simulink model "ForwardKinematicsSim2"  (R2020a)
settings: Solver=VariableStepAuto  StartTime=0.0  StopTime=10.0  RelTol=1e-3
settings Model: Creator=Sheldon  LastModifiedBy=alan

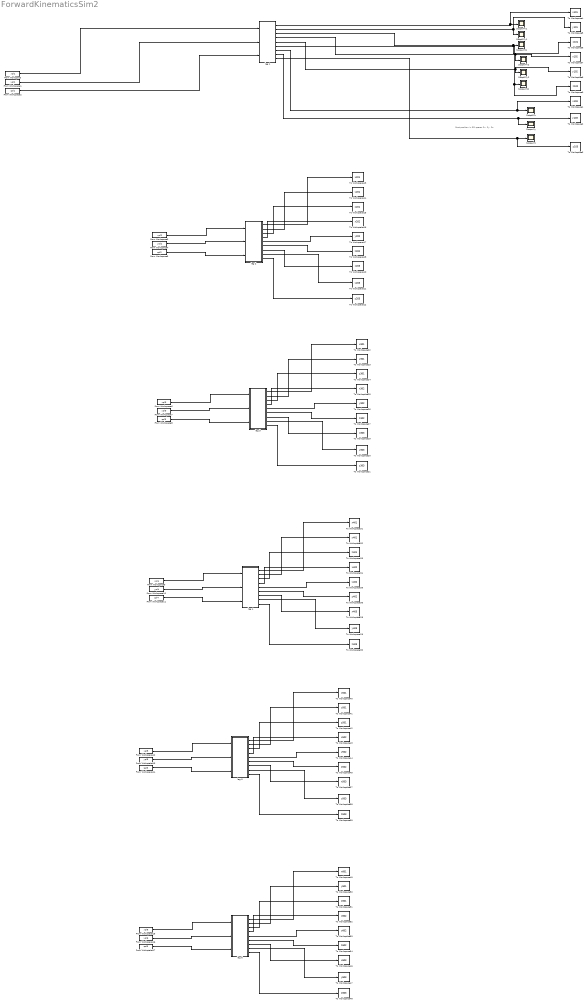
== system ForwardKinematicsSim2 ==
  note: Foot position in 3D space:
      | Px, Py, Pz
  From Workspace : FromWorkspace  VariableName=xpl1  SampleTime=1
  From Workspace1 : FromWorkspace  VariableName=ypl1  SampleTime=1
  From Workspace10 : FromWorkspace  VariableName=ypl4  SampleTime=1
  From Workspace11 : FromWorkspace  VariableName=zpl4  SampleTime=1
  From Workspace12 : FromWorkspace  VariableName=xpl5  SampleTime=1
  From Workspace13 : FromWorkspace  VariableName=ypl5  SampleTime=1
  From Workspace14 : FromWorkspace  VariableName=zpl5  SampleTime=1
  From Workspace15 : FromWorkspace  VariableName=xpl6  SampleTime=1
  From Workspace16 : FromWorkspace  VariableName=ypl6  SampleTime=1
  From Workspace17 : FromWorkspace  VariableName=zpl6  SampleTime=1
  From Workspace2 : FromWorkspace  VariableName=zpl1  SampleTime=1
  From Workspace3 : FromWorkspace  VariableName=xpl2  SampleTime=1
  From Workspace4 : FromWorkspace  VariableName=ypl2  SampleTime=1
  From Workspace5 : FromWorkspace  VariableName=zpl2  SampleTime=1
  From Workspace6 : FromWorkspace  VariableName=xpl3  SampleTime=1
  From Workspace7 : FromWorkspace  VariableName=ypl3  SampleTime=1
  From Workspace8 : FromWorkspace  VariableName=zpl3  SampleTime=1
  From Workspace9 : FromWorkspace  VariableName=xpl4  SampleTime=1
  Scope Px : Scope
  Scope Px1 : Scope
  Scope Px2 : Scope
  Scope Py : Scope
  Scope Py1 : Scope
  Scope Py2 : Scope
  Scope Pz : Scope
  Scope Pz1 : Scope
  Scope Pz2 : Scope
  To Workspace1 : ToWorkspace  VariableName=x103  SampleTime=-1
      settings: Save2DSignal=2-D array (concatenate along first dimension)
  To Workspace10 : ToWorkspace  VariableName=x203  SampleTime=-1
      settings: Save2DSignal=2-D array (concatenate along first dimension)
  To Workspace11 : ToWorkspace  VariableName=y203  SampleTime=-1
      settings: Save2DSignal=2-D array (concatenate along first dimension)
  To Workspace12 : ToWorkspace  VariableName=z203  SampleTime=-1
      settings: Save2DSignal=2-D array (concatenate along first dimension)
  To Workspace13 : ToWorkspace  VariableName=x201  SampleTime=-1
      settings: Save2DSignal=2-D array (concatenate along first dimension)
  To Workspace14 : ToWorkspace  VariableName=y201  SampleTime=-1
      settings: Save2DSignal=2-D array (concatenate along first dimension)
  To Workspace15 : ToWorkspace  VariableName=z201  SampleTime=-1
      settings: Save2DSignal=2-D array (concatenate along first dimension)
  To Workspace16 : ToWorkspace  VariableName=x202  SampleTime=-1
      settings: Save2DSignal=2-D array (concatenate along first dimension)
  To Workspace17 : ToWorkspace  VariableName=y202  SampleTime=-1
      settings: Save2DSignal=2-D array (concatenate along first dimension)
  To Workspace18 : ToWorkspace  VariableName=z202  SampleTime=-1
      settings: Save2DSignal=2-D array (concatenate along first dimension)
  To Workspace19 : ToWorkspace  VariableName=x303  SampleTime=-1
      settings: Save2DSignal=2-D array (concatenate along first dimension)
  To Workspace2 : ToWorkspace  VariableName=y103  SampleTime=-1
      settings: Save2DSignal=2-D array (concatenate along first dimension)
  To Workspace20 : ToWorkspace  VariableName=y303  SampleTime=-1
      settings: Save2DSignal=2-D array (concatenate along first dimension)
  To Workspace21 : ToWorkspace  VariableName=z303  SampleTime=-1
      settings: Save2DSignal=2-D array (concatenate along first dimension)
  To Workspace22 : ToWorkspace  VariableName=x301  SampleTime=-1
      settings: Save2DSignal=2-D array (concatenate along first dimension)
  To Workspace23 : ToWorkspace  VariableName=y301  SampleTime=-1
      settings: Save2DSignal=2-D array (concatenate along first dimension)
  To Workspace24 : ToWorkspace  VariableName=z301  SampleTime=-1
      settings: Save2DSignal=2-D array (concatenate along first dimension)
  To Workspace25 : ToWorkspace  VariableName=x302  SampleTime=-1
      settings: Save2DSignal=2-D array (concatenate along first dimension)
  To Workspace26 : ToWorkspace  VariableName=y302  SampleTime=-1
      settings: Save2DSignal=2-D array (concatenate along first dimension)
  To Workspace27 : ToWorkspace  VariableName=z302  SampleTime=-1
      settings: Save2DSignal=2-D array (concatenate along first dimension)
  To Workspace28 : ToWorkspace  VariableName=x403  SampleTime=-1
      settings: Save2DSignal=2-D array (concatenate along first dimension)
  To Workspace29 : ToWorkspace  VariableName=y403  SampleTime=-1
      settings: Save2DSignal=2-D array (concatenate along first dimension)
  To Workspace3 : ToWorkspace  VariableName=z103  SampleTime=-1
      settings: Save2DSignal=2-D array (concatenate along first dimension)
  To Workspace30 : ToWorkspace  VariableName=z403  SampleTime=-1
      settings: Save2DSignal=2-D array (concatenate along first dimension)
  To Workspace31 : ToWorkspace  VariableName=x401  SampleTime=-1
      settings: Save2DSignal=2-D array (concatenate along first dimension)
  To Workspace32 : ToWorkspace  VariableName=y401  SampleTime=-1
      settings: Save2DSignal=2-D array (concatenate along first dimension)
  To Workspace33 : ToWorkspace  VariableName=z401  SampleTime=-1
      settings: Save2DSignal=2-D array (concatenate along first dimension)
  To Workspace34 : ToWorkspace  VariableName=x402  SampleTime=-1
      settings: Save2DSignal=2-D array (concatenate along first dimension)
  To Workspace35 : ToWorkspace  VariableName=y402  SampleTime=-1
      settings: Save2DSignal=2-D array (concatenate along first dimension)
  To Workspace36 : ToWorkspace  VariableName=z402  SampleTime=-1
      settings: Save2DSignal=2-D array (concatenate along first dimension)
  To Workspace37 : ToWorkspace  VariableName=x503  SampleTime=-1
      settings: Save2DSignal=2-D array (concatenate along first dimension)
  To Workspace38 : ToWorkspace  VariableName=y503  SampleTime=-1
      settings: Save2DSignal=2-D array (concatenate along first dimension)
  To Workspace39 : ToWorkspace  VariableName=z503  SampleTime=-1
      settings: Save2DSignal=2-D array (concatenate along first dimension)
  To Workspace4 : ToWorkspace  VariableName=x101  SampleTime=-1
      settings: Save2DSignal=2-D array (concatenate along first dimension)
  To Workspace40 : ToWorkspace  VariableName=x501  SampleTime=-1
      settings: Save2DSignal=2-D array (concatenate along first dimension)
  To Workspace41 : ToWorkspace  VariableName=y501  SampleTime=-1
      settings: Save2DSignal=2-D array (concatenate along first dimension)
  To Workspace42 : ToWorkspace  VariableName=z501  SampleTime=-1
      settings: Save2DSignal=2-D array (concatenate along first dimension)
  To Workspace43 : ToWorkspace  VariableName=x502  SampleTime=-1
      settings: Save2DSignal=2-D array (concatenate along first dimension)
  To Workspace44 : ToWorkspace  VariableName=y502  SampleTime=-1
      settings: Save2DSignal=2-D array (concatenate along first dimension)
  To Workspace45 : ToWorkspace  VariableName=z502  SampleTime=-1
      settings: Save2DSignal=2-D array (concatenate along first dimension)
  To Workspace46 : ToWorkspace  VariableName=x603  SampleTime=-1
      settings: Save2DSignal=2-D array (concatenate along first dimension)
  To Workspace47 : ToWorkspace  VariableName=y603  SampleTime=-1
      settings: Save2DSignal=2-D array (concatenate along first dimension)
  To Workspace48 : ToWorkspace  VariableName=z603  SampleTime=-1
      settings: Save2DSignal=2-D array (concatenate along first dimension)
  To Workspace49 : ToWorkspace  VariableName=x601  SampleTime=-1
      settings: Save2DSignal=2-D array (concatenate along first dimension)
  To Workspace5 : ToWorkspace  VariableName=y101  SampleTime=-1
      settings: Save2DSignal=2-D array (concatenate along first dimension)
  To Workspace50 : ToWorkspace  VariableName=y601  SampleTime=-1
      settings: Save2DSignal=2-D array (concatenate along first dimension)
  To Workspace51 : ToWorkspace  VariableName=z601  SampleTime=-1
      settings: Save2DSignal=2-D array (concatenate along first dimension)
  To Workspace52 : ToWorkspace  VariableName=x602  SampleTime=-1
      settings: Save2DSignal=2-D array (concatenate along first dimension)
  To Workspace53 : ToWorkspace  VariableName=y602  SampleTime=-1
      settings: Save2DSignal=2-D array (concatenate along first dimension)
  To Workspace54 : ToWorkspace  VariableName=z602  SampleTime=-1
      settings: Save2DSignal=2-D array (concatenate along first dimension)
  To Workspace6 : ToWorkspace  VariableName=z101  SampleTime=-1
      settings: Save2DSignal=2-D array (concatenate along first dimension)
  To Workspace7 : ToWorkspace  VariableName=x102  SampleTime=-1
      settings: Save2DSignal=2-D array (concatenate along first dimension)
  To Workspace8 : ToWorkspace  VariableName=y102  SampleTime=-1
      settings: Save2DSignal=2-D array (concatenate along first dimension)
  To Workspace9 : ToWorkspace  VariableName=z102  SampleTime=-1
      settings: Save2DSignal=2-D array (concatenate along first dimension)
  leg 1 : Subsystem
  leg 2 : Subsystem
  leg 3 : Subsystem
  leg 4 : Subsystem
  leg 5 : Subsystem
  leg 6 : Subsystem
  wires:
  leg 1/6(Pz2) -> To Workspace9/1, Scope Pz2/1
  leg 1/5(Py2) -> Scope Py2/1, To Workspace8/1
  leg 1/1(Px1) -> To Workspace4/1, Scope Px1/1
  leg 1/9(Pz) -> To Workspace3/1, Scope Pz/1
  leg 1/3(Pz1) -> To Workspace6/1, Scope Pz1/1
  leg 1/2(Py1) -> Scope Py1/1, To Workspace5/1
  leg 1/7(Px) -> To Workspace1/1, Scope Px/1
  leg 1/4(Px2) -> Scope Px2/1, To Workspace7/1
  leg 1/8(Py) -> Scope Py/1, To Workspace2/1
  From Workspace/1 -> leg 1/1(xL)
  From Workspace1/1 -> leg 1/2(yL)
  From Workspace2/1 -> leg 1/3(zL)
  From Workspace3/1 -> leg 2/1(xL)
  From Workspace4/1 -> leg 2/2(yL)
  From Workspace5/1 -> leg 2/3(zL)
  leg 2/1(Px1) -> To Workspace13/1
  leg 2/2(Py1) -> To Workspace14/1
  leg 2/3(Pz1) -> To Workspace15/1
  leg 2/4(Px2) -> To Workspace16/1
  leg 2/5(Py2) -> To Workspace17/1
  leg 2/6(Pz2) -> To Workspace18/1
  leg 2/7(Px) -> To Workspace10/1
  leg 2/8(Py) -> To Workspace11/1
  leg 2/9(Pz) -> To Workspace12/1
  leg 3/7(Px) -> To Workspace19/1
  leg 3/4(Px2) -> To Workspace25/1
  leg 3/1(Px1) -> To Workspace22/1
  leg 3/5(Py2) -> To Workspace26/1
  From Workspace7/1 -> leg 3/2(yL)
  leg 3/3(Pz1) -> To Workspace24/1
  leg 3/9(Pz) -> To Workspace21/1
  leg 3/6(Pz2) -> To Workspace27/1
  leg 3/8(Py) -> To Workspace20/1
  From Workspace8/1 -> leg 3/3(zL)
  From Workspace6/1 -> leg 3/1(xL)
  leg 3/2(Py1) -> To Workspace23/1
  leg 4/7(Px) -> To Workspace28/1
  leg 4/4(Px2) -> To Workspace34/1
  leg 4/1(Px1) -> To Workspace31/1
  leg 4/5(Py2) -> To Workspace35/1
  From Workspace10/1 -> leg 4/2(yL)
  leg 4/3(Pz1) -> To Workspace33/1
  leg 4/9(Pz) -> To Workspace30/1
  leg 4/6(Pz2) -> To Workspace36/1
  leg 4/8(Py) -> To Workspace29/1
  From Workspace11/1 -> leg 4/3(zL)
  From Workspace9/1 -> leg 4/1(xL)
  leg 4/2(Py1) -> To Workspace32/1
  leg 5/7(Px) -> To Workspace37/1
  leg 5/4(Px2) -> To Workspace43/1
  leg 5/1(Px1) -> To Workspace40/1
  leg 5/5(Py2) -> To Workspace44/1
  From Workspace13/1 -> leg 5/2(yL)
  leg 5/3(Pz1) -> To Workspace42/1
  leg 5/9(Pz) -> To Workspace39/1
  leg 5/6(Pz2) -> To Workspace45/1
  leg 5/8(Py) -> To Workspace38/1
  From Workspace14/1 -> leg 5/3(zL)
  From Workspace12/1 -> leg 5/1(xL)
  leg 5/2(Py1) -> To Workspace41/1
  leg 6/7(Px) -> To Workspace46/1
  leg 6/4(Px2) -> To Workspace52/1
  leg 6/1(Px1) -> To Workspace49/1
  leg 6/5(Py2) -> To Workspace53/1
  From Workspace16/1 -> leg 6/2(yL)
  leg 6/3(Pz1) -> To Workspace51/1
  leg 6/9(Pz) -> To Workspace48/1
  leg 6/6(Pz2) -> To Workspace54/1
  leg 6/8(Py) -> To Workspace47/1
  From Workspace17/1 -> leg 6/3(zL)
  From Workspace15/1 -> leg 6/1(xL)
  leg 6/2(Py1) -> To Workspace50/1

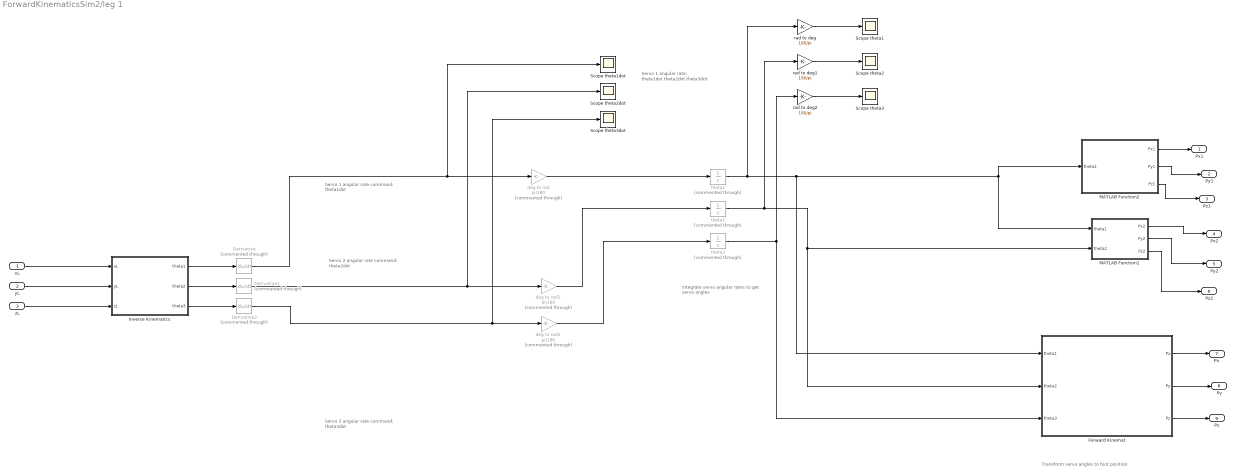
== system ForwardKinematicsSim2/leg 1 ==
  note: Servo 1 angular rate:
      |
      | theta1dot
      | theta2dot
      | theta3dot
  note: Servo 1 angular rate
      | command: theta1dot
  note: Servo 2 angular rate
      | command: theta2dot
  note: Integrate servo angular rates to get servo angles
  note: Servo 3 angular rate
      | command: theta3dot
  note: Transform servo angles to foot position
  xL : Inport
  yL : Inport  Port=2
  zL : Inport  Port=3
  Derivative : Derivative  Commented=through
  Derivative1 : Derivative  Commented=through
  Derivative2 : Derivative  Commented=through
  Forward Kinemat : MATLAB Function  TreatAsAtomicUnit=on
  Inverse Kinematics : MATLAB Function  TreatAsAtomicUnit=on
  MATLAB Function1 : MATLAB Function  TreatAsAtomicUnit=on
  MATLAB Function2 : MATLAB Function  TreatAsAtomicUnit=on
  Scope theta1 : Scope
  Scope theta1dot : Scope
  Scope theta2 : Scope
  Scope theta2dot : Scope
  Scope theta3 : Scope
  Scope theta3dot : Scope
  deg to rad : Gain  Commented=through  Gain=pi/180
  deg to rad1 : Gain  Commented=through  Gain=pi/180
  deg to rad2 : Gain  Commented=through  Gain=pi/180
  rad to deg : Gain  Gain=180/pi
  rad to deg1 : Gain  Gain=180/pi
  rad to deg2 : Gain  Gain=180/pi
  theta1 : Integrator  Commented=through
  theta2 : Integrator  Commented=through
  theta3 : Integrator  Commented=through
  Px1 : Outport
  Py1 : Outport  Port=2
  Pz1 : Outport  Port=3
  Px2 : Outport  Port=4
  Py2 : Outport  Port=5
  Pz2 : Outport  Port=6
  Px : Outport  Port=7
  Py : Outport  Port=8
  Pz : Outport  Port=9
  wires:
  deg to rad/1 -> theta1/1
  rad to deg1/1 -> Scope theta2/1
  theta1/1 -> MATLAB Function1/1(theta1), MATLAB Function2/1(theta1), Forward Kinemat/1(theta1), rad to deg/1
  Derivative/1 -> Scope theta1dot/1, deg to rad/1
  theta2/1 -> MATLAB Function1/2(theta2), Forward Kinemat/2(theta2), rad to deg1/1
  deg to rad2/1 -> theta3/1
  Inverse Kinematics/1(theta1) -> Derivative/1
  rad to deg2/1 -> Scope theta3/1
  Inverse Kinematics/2(theta2) -> Derivative1/1
  MATLAB Function2/2(Py1) -> Py1/1
  deg to rad1/1 -> theta2/1
  theta3/1 -> rad to deg2/1, Forward Kinemat/3(theta3)
  Inverse Kinematics/3(theta3) -> Derivative2/1
  MATLAB Function1/1(Px2) -> Px2/1
  Derivative2/1 -> Scope theta3dot/1, deg to rad2/1
  Derivative1/1 -> deg to rad1/1, Scope theta2dot/1
  rad to deg/1 -> Scope theta1/1
  zL/1 -> Inverse Kinematics/3(zL)
  Forward Kinemat/1(Px) -> Px/1
  Forward Kinemat/2(Py) -> Py/1
  Forward Kinemat/3(Pz) -> Pz/1
  MATLAB Function2/3(Pz1) -> Pz1/1
  MATLAB Function2/1(Px1) -> Px1/1
  MATLAB Function1/2(Py2) -> Py2/1
  yL/1 -> Inverse Kinematics/2(yL)
  MATLAB Function1/3(Pz2) -> Pz2/1
  xL/1 -> Inverse Kinematics/1(xL)

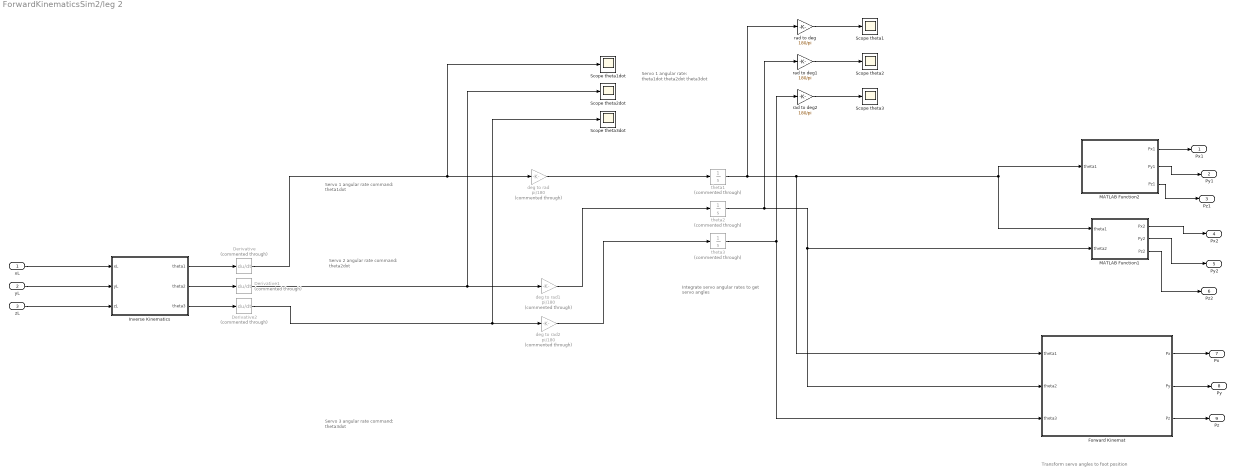
== system ForwardKinematicsSim2/leg 2 ==
  note: Servo 1 angular rate:
      |
      | theta1dot
      | theta2dot
      | theta3dot
  note: Servo 1 angular rate
      | command: theta1dot
  note: Servo 2 angular rate
      | command: theta2dot
  note: Integrate servo angular rates to get servo angles
  note: Servo 3 angular rate
      | command: theta3dot
  note: Transform servo angles to foot position
  xL : Inport
  yL : Inport  Port=2
  zL : Inport  Port=3
  Derivative : Derivative  Commented=through
  Derivative1 : Derivative  Commented=through
  Derivative2 : Derivative  Commented=through
  Forward Kinemat : MATLAB Function  TreatAsAtomicUnit=on
  Inverse Kinematics : MATLAB Function  TreatAsAtomicUnit=on
  MATLAB Function1 : MATLAB Function  TreatAsAtomicUnit=on
  MATLAB Function2 : MATLAB Function  TreatAsAtomicUnit=on
  Scope theta1 : Scope
  Scope theta1dot : Scope
  Scope theta2 : Scope
  Scope theta2dot : Scope
  Scope theta3 : Scope
  Scope theta3dot : Scope
  deg to rad : Gain  Commented=through  Gain=pi/180
  deg to rad1 : Gain  Commented=through  Gain=pi/180
  deg to rad2 : Gain  Commented=through  Gain=pi/180
  rad to deg : Gain  Gain=180/pi
  rad to deg1 : Gain  Gain=180/pi
  rad to deg2 : Gain  Gain=180/pi
  theta1 : Integrator  Commented=through
  theta2 : Integrator  Commented=through
  theta3 : Integrator  Commented=through
  Px1 : Outport
  Py1 : Outport  Port=2
  Pz1 : Outport  Port=3
  Px2 : Outport  Port=4
  Py2 : Outport  Port=5
  Pz2 : Outport  Port=6
  Px : Outport  Port=7
  Py : Outport  Port=8
  Pz : Outport  Port=9
  wires:
  deg to rad/1 -> theta1/1
  rad to deg1/1 -> Scope theta2/1
  theta1/1 -> MATLAB Function1/1(theta1), MATLAB Function2/1(theta1), Forward Kinemat/1(theta1), rad to deg/1
  Derivative/1 -> Scope theta1dot/1, deg to rad/1
  theta2/1 -> MATLAB Function1/2(theta2), Forward Kinemat/2(theta2), rad to deg1/1
  deg to rad2/1 -> theta3/1
  Inverse Kinematics/1(theta1) -> Derivative/1
  rad to deg2/1 -> Scope theta3/1
  Inverse Kinematics/2(theta2) -> Derivative1/1
  MATLAB Function2/2(Py1) -> Py1/1
  deg to rad1/1 -> theta2/1
  theta3/1 -> rad to deg2/1, Forward Kinemat/3(theta3)
  Inverse Kinematics/3(theta3) -> Derivative2/1
  MATLAB Function1/1(Px2) -> Px2/1
  Derivative2/1 -> Scope theta3dot/1, deg to rad2/1
  Derivative1/1 -> deg to rad1/1, Scope theta2dot/1
  rad to deg/1 -> Scope theta1/1
  zL/1 -> Inverse Kinematics/3(zL)
  Forward Kinemat/1(Px) -> Px/1
  Forward Kinemat/2(Py) -> Py/1
  Forward Kinemat/3(Pz) -> Pz/1
  MATLAB Function2/3(Pz1) -> Pz1/1
  MATLAB Function2/1(Px1) -> Px1/1
  MATLAB Function1/2(Py2) -> Py2/1
  yL/1 -> Inverse Kinematics/2(yL)
  MATLAB Function1/3(Pz2) -> Pz2/1
  xL/1 -> Inverse Kinematics/1(xL)

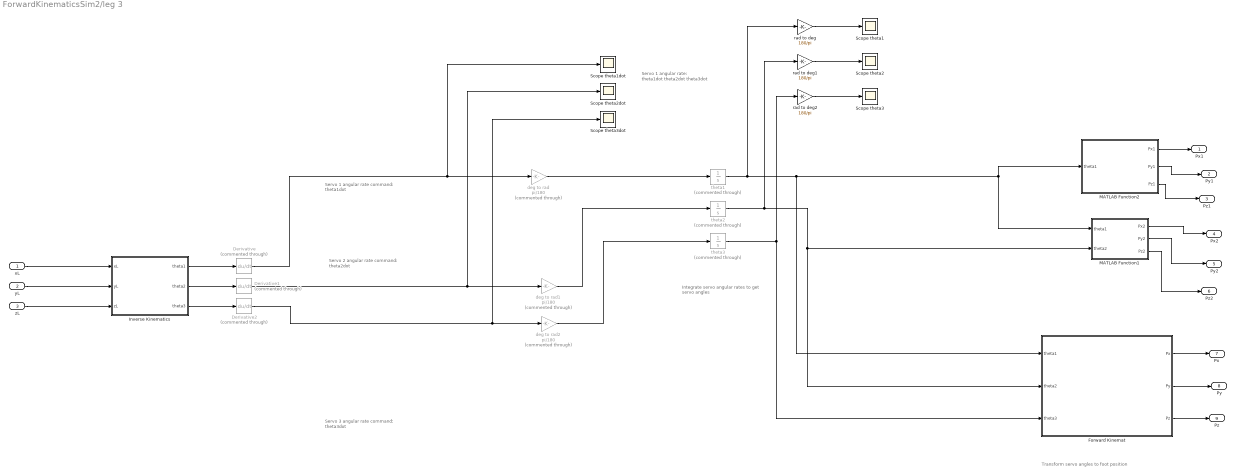
== system ForwardKinematicsSim2/leg 3 ==
  note: Servo 1 angular rate:
      |
      | theta1dot
      | theta2dot
      | theta3dot
  note: Servo 1 angular rate
      | command: theta1dot
  note: Servo 2 angular rate
      | command: theta2dot
  note: Integrate servo angular rates to get servo angles
  note: Servo 3 angular rate
      | command: theta3dot
  note: Transform servo angles to foot position
  xL : Inport
  yL : Inport  Port=2
  zL : Inport  Port=3
  Derivative : Derivative  Commented=through
  Derivative1 : Derivative  Commented=through
  Derivative2 : Derivative  Commented=through
  Forward Kinemat : MATLAB Function  TreatAsAtomicUnit=on
  Inverse Kinematics : MATLAB Function  TreatAsAtomicUnit=on
  MATLAB Function1 : MATLAB Function  TreatAsAtomicUnit=on
  MATLAB Function2 : MATLAB Function  TreatAsAtomicUnit=on
  Scope theta1 : Scope
  Scope theta1dot : Scope
  Scope theta2 : Scope
  Scope theta2dot : Scope
  Scope theta3 : Scope
  Scope theta3dot : Scope
  deg to rad : Gain  Commented=through  Gain=pi/180
  deg to rad1 : Gain  Commented=through  Gain=pi/180
  deg to rad2 : Gain  Commented=through  Gain=pi/180
  rad to deg : Gain  Gain=180/pi
  rad to deg1 : Gain  Gain=180/pi
  rad to deg2 : Gain  Gain=180/pi
  theta1 : Integrator  Commented=through
  theta2 : Integrator  Commented=through
  theta3 : Integrator  Commented=through
  Px1 : Outport
  Py1 : Outport  Port=2
  Pz1 : Outport  Port=3
  Px2 : Outport  Port=4
  Py2 : Outport  Port=5
  Pz2 : Outport  Port=6
  Px : Outport  Port=7
  Py : Outport  Port=8
  Pz : Outport  Port=9
  wires:
  deg to rad/1 -> theta1/1
  rad to deg1/1 -> Scope theta2/1
  theta1/1 -> MATLAB Function1/1(theta1), MATLAB Function2/1(theta1), Forward Kinemat/1(theta1), rad to deg/1
  Derivative/1 -> Scope theta1dot/1, deg to rad/1
  theta2/1 -> MATLAB Function1/2(theta2), Forward Kinemat/2(theta2), rad to deg1/1
  deg to rad2/1 -> theta3/1
  Inverse Kinematics/1(theta1) -> Derivative/1
  rad to deg2/1 -> Scope theta3/1
  Inverse Kinematics/2(theta2) -> Derivative1/1
  MATLAB Function2/2(Py1) -> Py1/1
  deg to rad1/1 -> theta2/1
  theta3/1 -> rad to deg2/1, Forward Kinemat/3(theta3)
  Inverse Kinematics/3(theta3) -> Derivative2/1
  MATLAB Function1/1(Px2) -> Px2/1
  Derivative2/1 -> Scope theta3dot/1, deg to rad2/1
  Derivative1/1 -> deg to rad1/1, Scope theta2dot/1
  rad to deg/1 -> Scope theta1/1
  zL/1 -> Inverse Kinematics/3(zL)
  Forward Kinemat/1(Px) -> Px/1
  Forward Kinemat/2(Py) -> Py/1
  Forward Kinemat/3(Pz) -> Pz/1
  MATLAB Function2/3(Pz1) -> Pz1/1
  MATLAB Function2/1(Px1) -> Px1/1
  MATLAB Function1/2(Py2) -> Py2/1
  yL/1 -> Inverse Kinematics/2(yL)
  MATLAB Function1/3(Pz2) -> Pz2/1
  xL/1 -> Inverse Kinematics/1(xL)

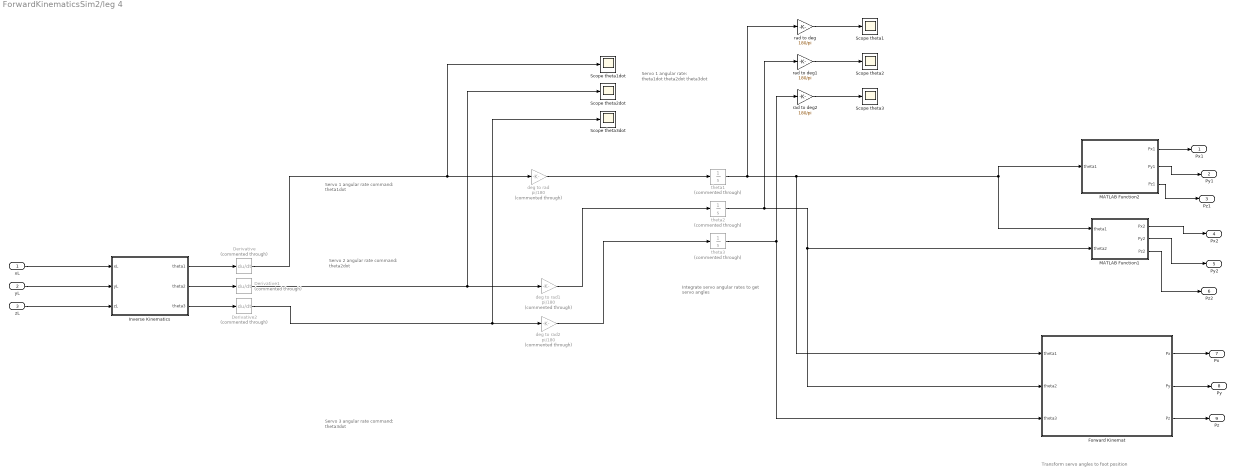
== system ForwardKinematicsSim2/leg 4 ==
  note: Servo 1 angular rate:
      |
      | theta1dot
      | theta2dot
      | theta3dot
  note: Servo 1 angular rate
      | command: theta1dot
  note: Servo 2 angular rate
      | command: theta2dot
  note: Integrate servo angular rates to get servo angles
  note: Servo 3 angular rate
      | command: theta3dot
  note: Transform servo angles to foot position
  xL : Inport
  yL : Inport  Port=2
  zL : Inport  Port=3
  Derivative : Derivative  Commented=through
  Derivative1 : Derivative  Commented=through
  Derivative2 : Derivative  Commented=through
  Forward Kinemat : MATLAB Function  TreatAsAtomicUnit=on
  Inverse Kinematics : MATLAB Function  TreatAsAtomicUnit=on
  MATLAB Function1 : MATLAB Function  TreatAsAtomicUnit=on
  MATLAB Function2 : MATLAB Function  TreatAsAtomicUnit=on
  Scope theta1 : Scope
  Scope theta1dot : Scope
  Scope theta2 : Scope
  Scope theta2dot : Scope
  Scope theta3 : Scope
  Scope theta3dot : Scope
  deg to rad : Gain  Commented=through  Gain=pi/180
  deg to rad1 : Gain  Commented=through  Gain=pi/180
  deg to rad2 : Gain  Commented=through  Gain=pi/180
  rad to deg : Gain  Gain=180/pi
  rad to deg1 : Gain  Gain=180/pi
  rad to deg2 : Gain  Gain=180/pi
  theta1 : Integrator  Commented=through
  theta2 : Integrator  Commented=through
  theta3 : Integrator  Commented=through
  Px1 : Outport
  Py1 : Outport  Port=2
  Pz1 : Outport  Port=3
  Px2 : Outport  Port=4
  Py2 : Outport  Port=5
  Pz2 : Outport  Port=6
  Px : Outport  Port=7
  Py : Outport  Port=8
  Pz : Outport  Port=9
  wires:
  deg to rad/1 -> theta1/1
  rad to deg1/1 -> Scope theta2/1
  theta1/1 -> MATLAB Function1/1(theta1), MATLAB Function2/1(theta1), Forward Kinemat/1(theta1), rad to deg/1
  Derivative/1 -> Scope theta1dot/1, deg to rad/1
  theta2/1 -> MATLAB Function1/2(theta2), Forward Kinemat/2(theta2), rad to deg1/1
  deg to rad2/1 -> theta3/1
  Inverse Kinematics/1(theta1) -> Derivative/1
  rad to deg2/1 -> Scope theta3/1
  Inverse Kinematics/2(theta2) -> Derivative1/1
  MATLAB Function2/2(Py1) -> Py1/1
  deg to rad1/1 -> theta2/1
  theta3/1 -> rad to deg2/1, Forward Kinemat/3(theta3)
  Inverse Kinematics/3(theta3) -> Derivative2/1
  MATLAB Function1/1(Px2) -> Px2/1
  Derivative2/1 -> Scope theta3dot/1, deg to rad2/1
  Derivative1/1 -> deg to rad1/1, Scope theta2dot/1
  rad to deg/1 -> Scope theta1/1
  zL/1 -> Inverse Kinematics/3(zL)
  Forward Kinemat/1(Px) -> Px/1
  Forward Kinemat/2(Py) -> Py/1
  Forward Kinemat/3(Pz) -> Pz/1
  MATLAB Function2/3(Pz1) -> Pz1/1
  MATLAB Function2/1(Px1) -> Px1/1
  MATLAB Function1/2(Py2) -> Py2/1
  yL/1 -> Inverse Kinematics/2(yL)
  MATLAB Function1/3(Pz2) -> Pz2/1
  xL/1 -> Inverse Kinematics/1(xL)

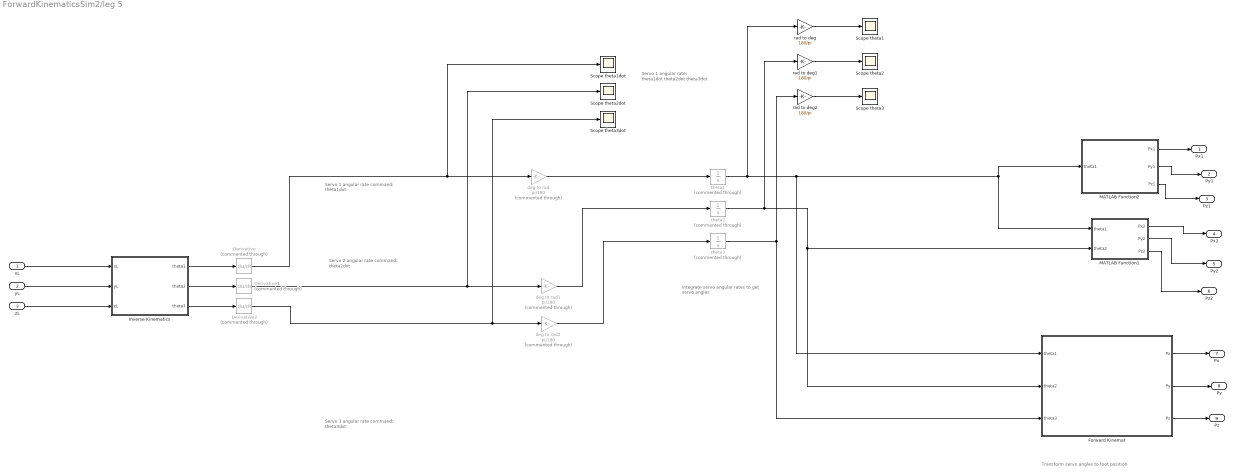
== system ForwardKinematicsSim2/leg 5 ==
  note: Servo 1 angular rate:
      |
      | theta1dot
      | theta2dot
      | theta3dot
  note: Servo 1 angular rate
      | command: theta1dot
  note: Servo 2 angular rate
      | command: theta2dot
  note: Integrate servo angular rates to get servo angles
  note: Servo 3 angular rate
      | command: theta3dot
  note: Transform servo angles to foot position
  xL : Inport
  yL : Inport  Port=2
  zL : Inport  Port=3
  Derivative : Derivative  Commented=through
  Derivative1 : Derivative  Commented=through
  Derivative2 : Derivative  Commented=through
  Forward Kinemat : MATLAB Function  TreatAsAtomicUnit=on
  Inverse Kinematics : MATLAB Function  TreatAsAtomicUnit=on
  MATLAB Function1 : MATLAB Function  TreatAsAtomicUnit=on
  MATLAB Function2 : MATLAB Function  TreatAsAtomicUnit=on
  Scope theta1 : Scope
  Scope theta1dot : Scope
  Scope theta2 : Scope
  Scope theta2dot : Scope
  Scope theta3 : Scope
  Scope theta3dot : Scope
  deg to rad : Gain  Commented=through  Gain=pi/180
  deg to rad1 : Gain  Commented=through  Gain=pi/180
  deg to rad2 : Gain  Commented=through  Gain=pi/180
  rad to deg : Gain  Gain=180/pi
  rad to deg1 : Gain  Gain=180/pi
  rad to deg2 : Gain  Gain=180/pi
  theta1 : Integrator  Commented=through
  theta2 : Integrator  Commented=through
  theta3 : Integrator  Commented=through
  Px1 : Outport
  Py1 : Outport  Port=2
  Pz1 : Outport  Port=3
  Px2 : Outport  Port=4
  Py2 : Outport  Port=5
  Pz2 : Outport  Port=6
  Px : Outport  Port=7
  Py : Outport  Port=8
  Pz : Outport  Port=9
  wires:
  deg to rad/1 -> theta1/1
  rad to deg1/1 -> Scope theta2/1
  theta1/1 -> MATLAB Function1/1(theta1), MATLAB Function2/1(theta1), Forward Kinemat/1(theta1), rad to deg/1
  Derivative/1 -> Scope theta1dot/1, deg to rad/1
  theta2/1 -> MATLAB Function1/2(theta2), Forward Kinemat/2(theta2), rad to deg1/1
  deg to rad2/1 -> theta3/1
  Inverse Kinematics/1(theta1) -> Derivative/1
  rad to deg2/1 -> Scope theta3/1
  Inverse Kinematics/2(theta2) -> Derivative1/1
  MATLAB Function2/2(Py1) -> Py1/1
  deg to rad1/1 -> theta2/1
  theta3/1 -> rad to deg2/1, Forward Kinemat/3(theta3)
  Inverse Kinematics/3(theta3) -> Derivative2/1
  MATLAB Function1/1(Px2) -> Px2/1
  Derivative2/1 -> Scope theta3dot/1, deg to rad2/1
  Derivative1/1 -> deg to rad1/1, Scope theta2dot/1
  rad to deg/1 -> Scope theta1/1
  zL/1 -> Inverse Kinematics/3(zL)
  Forward Kinemat/1(Px) -> Px/1
  Forward Kinemat/2(Py) -> Py/1
  Forward Kinemat/3(Pz) -> Pz/1
  MATLAB Function2/3(Pz1) -> Pz1/1
  MATLAB Function2/1(Px1) -> Px1/1
  MATLAB Function1/2(Py2) -> Py2/1
  yL/1 -> Inverse Kinematics/2(yL)
  MATLAB Function1/3(Pz2) -> Pz2/1
  xL/1 -> Inverse Kinematics/1(xL)

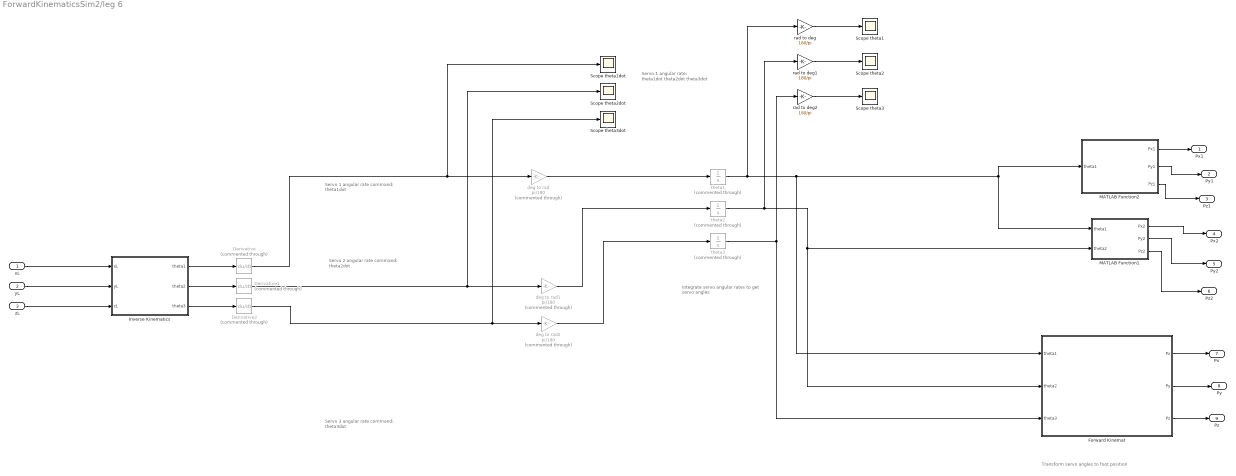
== system ForwardKinematicsSim2/leg 6 ==
  note: Servo 1 angular rate:
      |
      | theta1dot
      | theta2dot
      | theta3dot
  note: Servo 1 angular rate
      | command: theta1dot
  note: Servo 2 angular rate
      | command: theta2dot
  note: Integrate servo angular rates to get servo angles
  note: Servo 3 angular rate
      | command: theta3dot
  note: Transform servo angles to foot position
  xL : Inport
  yL : Inport  Port=2
  zL : Inport  Port=3
  Derivative : Derivative  Commented=through
  Derivative1 : Derivative  Commented=through
  Derivative2 : Derivative  Commented=through
  Forward Kinemat : MATLAB Function  TreatAsAtomicUnit=on
  Inverse Kinematics : MATLAB Function  TreatAsAtomicUnit=on
  MATLAB Function1 : MATLAB Function  TreatAsAtomicUnit=on
  MATLAB Function2 : MATLAB Function  TreatAsAtomicUnit=on
  Scope theta1 : Scope
  Scope theta1dot : Scope
  Scope theta2 : Scope
  Scope theta2dot : Scope
  Scope theta3 : Scope
  Scope theta3dot : Scope
  deg to rad : Gain  Commented=through  Gain=pi/180
  deg to rad1 : Gain  Commented=through  Gain=pi/180
  deg to rad2 : Gain  Commented=through  Gain=pi/180
  rad to deg : Gain  Gain=180/pi
  rad to deg1 : Gain  Gain=180/pi
  rad to deg2 : Gain  Gain=180/pi
  theta1 : Integrator  Commented=through
  theta2 : Integrator  Commented=through
  theta3 : Integrator  Commented=through
  Px1 : Outport
  Py1 : Outport  Port=2
  Pz1 : Outport  Port=3
  Px2 : Outport  Port=4
  Py2 : Outport  Port=5
  Pz2 : Outport  Port=6
  Px : Outport  Port=7
  Py : Outport  Port=8
  Pz : Outport  Port=9
  wires:
  deg to rad/1 -> theta1/1
  rad to deg1/1 -> Scope theta2/1
  theta1/1 -> MATLAB Function1/1(theta1), MATLAB Function2/1(theta1), Forward Kinemat/1(theta1), rad to deg/1
  Derivative/1 -> Scope theta1dot/1, deg to rad/1
  theta2/1 -> MATLAB Function1/2(theta2), Forward Kinemat/2(theta2), rad to deg1/1
  deg to rad2/1 -> theta3/1
  Inverse Kinematics/1(theta1) -> Derivative/1
  rad to deg2/1 -> Scope theta3/1
  Inverse Kinematics/2(theta2) -> Derivative1/1
  MATLAB Function2/2(Py1) -> Py1/1
  deg to rad1/1 -> theta2/1
  theta3/1 -> rad to deg2/1, Forward Kinemat/3(theta3)
  Inverse Kinematics/3(theta3) -> Derivative2/1
  MATLAB Function1/1(Px2) -> Px2/1
  Derivative2/1 -> Scope theta3dot/1, deg to rad2/1
  Derivative1/1 -> deg to rad1/1, Scope theta2dot/1
  rad to deg/1 -> Scope theta1/1
  zL/1 -> Inverse Kinematics/3(zL)
  Forward Kinemat/1(Px) -> Px/1
  Forward Kinemat/2(Py) -> Py/1
  Forward Kinemat/3(Pz) -> Pz/1
  MATLAB Function2/3(Pz1) -> Pz1/1
  MATLAB Function2/1(Px1) -> Px1/1
  MATLAB Function1/2(Py2) -> Py2/1
  yL/1 -> Inverse Kinematics/2(yL)
  MATLAB Function1/3(Pz2) -> Pz2/1
  xL/1 -> Inverse Kinematics/1(xL)

== matlab function ForwardKinematicsSim2/leg 3/Inverse Kinematics ==
  data: xL input; theta1 output; yL input; zL input; theta2 output; theta3 output
function [theta1,theta2,theta3] = fcn(xL,yL,zL)
    
    L1x = 53.17;
    L1z = 8;
    L2  = 101.88;
    L3  = 149.16;

    theta1 = atan2(yL,xL);

    C1  = cos(theta1);
    S1  = sin(theta1);

    C3_temp = ( ( xL - L1x*C1 )^2 + ( yL - L1x*S1 )^2 + ( zL - L1z )^2 - L2^2 - L3^2 )/( 2*L2*L3 );
    
    if C3_temp>1
        C3 = 1;
    elseif C3_temp<-1
        C3 = -1;
    else
        C3 = C3_temp;
    end
    
    S3 = -sqrt((1 - C3^2));

    theta2 = atan2( zL-L1z, sqrt( (xL-L1x*C1)^2 + (yL - L1x*S1)^2 ) ) - atan2(L3*S3, L2 + L3*C3);

    theta3 = atan2(S3, C3);
    
end

== matlab function ForwardKinematicsSim2/leg 3/MATLAB Function1 ==
  data: theta1 input; Px2 output; theta2 input; Py2 output; Pz2 output
function [Px2,Py2,Pz2] = fcn(theta1,theta2)

    % Link lengths as defined in Figure 5.3
    L1x = 53.17;
    L1z = 8;
    L2  = 101.88;

    
    % Transformation from servo angles to end effector positions as given in
    % Equation 5.30
    C1  = cos(theta1);
    S1  = sin(theta1);
    C2  = cos(theta2);
    S2  = sin(theta2);
    
    H01 = [C1,  0,  S1, C1*L1x;...
           S1,  0, -C1, S1*L1x;...
            0,  1,   0,    L1z;...
            0,  0,   0,     1];
   
    H12 = [C2, -S2,  0, L2*C2;...
           S2,  C2,  0, L2*S2;...
            0,   0,  1,     0;...
            0,   0,  0,     1];  
    
    H02 = H01*H12;
 
Px2 = H02(1,4);Py2 = H02(2,4);Pz2 = H02(3,4);

== matlab function ForwardKinematicsSim2/leg 1/MATLAB Function1 ==
  data: theta1 input; Px2 output; theta2 input; Py2 output; Pz2 output
function [Px2,Py2,Pz2] = fcn(theta1,theta2)

    % Link lengths as defined in Figure 5.3
    L1x = 53.17;
    L1z = 8;
    L2  = 101.88;

    
    % Transformation from servo angles to end effector positions as given in
    % Equation 5.30
    C1  = cos(theta1);
    S1  = sin(theta1);
    C2  = cos(theta2);
    S2  = sin(theta2);
    
    H01 = [C1,  0,  S1, C1*L1x;...
           S1,  0, -C1, S1*L1x;...
            0,  1,   0,    L1z;...
            0,  0,   0,     1];
   
    H12 = [C2, -S2,  0, L2*C2;...
           S2,  C2,  0, L2*S2;...
            0,   0,  1,     0;...
            0,   0,  0,     1];  
    
    H02 = H01*H12;
 
Px2 = H02(1,4);Py2 = H02(2,4);Pz2 = H02(3,4);

== matlab function ForwardKinematicsSim2/leg 3/MATLAB Function2 ==
  data: theta1 input; Px1 output; Py1 output; Pz1 output
function [Px1,Py1,Pz1] = fcn(theta1)

    % Link lengths as defined in Figure 5.3
    L1x = 53.17;
    L1z = 8;

    % Transformation from servo angles to end effector positions as given in
    % Equation 5.30
    C1  = cos(theta1);
    S1  = sin(theta1);

    H01 = [C1,  0,  S1, C1*L1x;...
           S1,  0, -C1, S1*L1x;...
            0,  1,   0,    L1z;...
            0,  0,   0,     1];
 
Px1 = H01(1,4);Py1 = H01(2,4);Pz1 = H01(3,4);

== matlab function ForwardKinematicsSim2/leg 4/Forward Kinemat ==
  data: theta1 input; Px output; theta2 input; theta3 input; Py output; Pz output
function [Px,Py,Pz] = fcn(theta1,theta2,theta3)

    % degrees to radians
    d2r = pi/180;

    % Link lengths as defined in Figure 5.3
    L1x = 53.17;
    L1z = 8;
    L2  = 101.88;
    L3  = 149.16;

    % Transformation from servo angles to end effector positions as given in
    % Equation 5.30
    C1  = cos(theta1);
    S1  = sin(theta1);
    C2  = cos(theta2);
    S2  = sin(theta2);
    C23 = cos(theta2 + theta3);
    S23 = sin(theta2 + theta3);

    T03 = [C1*C23, -C1*S23,  S1, C1*(L1x + L3*C23 + L2*C2);...
            S1*C23, -S1*S23, -C1, S1*(L1x + L3*C23 + L2*C2);...
            S23,     C23,   0, L1z + L3*S23 + L2*S2;...
            0,       0,   0, 1];
 
Px = T03(1,4);Py = T03(2,4);Pz = T03(3,4);

== matlab function ForwardKinematicsSim2/leg 4/Inverse Kinematics ==
  data: xL input; theta1 output; yL input; zL input; theta2 output; theta3 output
function [theta1,theta2,theta3] = fcn(xL,yL,zL)
    
    L1x = 53.17;
    L1z = 8;
    L2  = 101.88;
    L3  = 149.16;

    theta1 = atan2(yL,xL);

    C1  = cos(theta1);
    S1  = sin(theta1);

    C3_temp = ( ( xL - L1x*C1 )^2 + ( yL - L1x*S1 )^2 + ( zL - L1z )^2 - L2^2 - L3^2 )/( 2*L2*L3 );
    
    if C3_temp>1
        C3 = 1;
    elseif C3_temp<-1
        C3 = -1;
    else
        C3 = C3_temp;
    end
    
    S3 = -sqrt((1 - C3^2));

    theta2 = atan2( zL-L1z, sqrt( (xL-L1x*C1)^2 + (yL - L1x*S1)^2 ) ) - atan2(L3*S3, L2 + L3*C3);

    theta3 = atan2(S3, C3);
    
end

== matlab function ForwardKinematicsSim2/leg 4/MATLAB Function1 ==
  data: theta1 input; Px2 output; theta2 input; Py2 output; Pz2 output
function [Px2,Py2,Pz2] = fcn(theta1,theta2)

    % Link lengths as defined in Figure 5.3
    L1x = 53.17;
    L1z = 8;
    L2  = 101.88;

    
    % Transformation from servo angles to end effector positions as given in
    % Equation 5.30
    C1  = cos(theta1);
    S1  = sin(theta1);
    C2  = cos(theta2);
    S2  = sin(theta2);
    
    H01 = [C1,  0,  S1, C1*L1x;...
           S1,  0, -C1, S1*L1x;...
            0,  1,   0,    L1z;...
            0,  0,   0,     1];
   
    H12 = [C2, -S2,  0, L2*C2;...
           S2,  C2,  0, L2*S2;...
            0,   0,  1,     0;...
            0,   0,  0,     1];  
    
    H02 = H01*H12;
 
Px2 = H02(1,4);Py2 = H02(2,4);Pz2 = H02(3,4);

== matlab function ForwardKinematicsSim2/leg 4/MATLAB Function2 ==
  data: theta1 input; Px1 output; Py1 output; Pz1 output
function [Px1,Py1,Pz1] = fcn(theta1)

    % Link lengths as defined in Figure 5.3
    L1x = 53.17;
    L1z = 8;

    % Transformation from servo angles to end effector positions as given in
    % Equation 5.30
    C1  = cos(theta1);
    S1  = sin(theta1);

    H01 = [C1,  0,  S1, C1*L1x;...
           S1,  0, -C1, S1*L1x;...
            0,  1,   0,    L1z;...
            0,  0,   0,     1];
 
Px1 = H01(1,4);Py1 = H01(2,4);Pz1 = H01(3,4);

== matlab function ForwardKinematicsSim2/leg 5/Forward Kinemat ==
  data: theta1 input; Px output; theta2 input; theta3 input; Py output; Pz output
function [Px,Py,Pz] = fcn(theta1,theta2,theta3)

    % degrees to radians
    d2r = pi/180;

    % Link lengths as defined in Figure 5.3
    L1x = 53.17;
    L1z = 8;
    L2  = 101.88;
    L3  = 149.16;

    % Transformation from servo angles to end effector positions as given in
    % Equation 5.30
    C1  = cos(theta1);
    S1  = sin(theta1);
    C2  = cos(theta2);
    S2  = sin(theta2);
    C23 = cos(theta2 + theta3);
    S23 = sin(theta2 + theta3);

    T03 = [C1*C23, -C1*S23,  S1, C1*(L1x + L3*C23 + L2*C2);...
            S1*C23, -S1*S23, -C1, S1*(L1x + L3*C23 + L2*C2);...
            S23,     C23,   0, L1z + L3*S23 + L2*S2;...
            0,       0,   0, 1];
 
Px = T03(1,4);Py = T03(2,4);Pz = T03(3,4);

== matlab function ForwardKinematicsSim2/leg 5/Inverse Kinematics ==
  data: xL input; theta1 output; yL input; zL input; theta2 output; theta3 output
function [theta1,theta2,theta3] = fcn(xL,yL,zL)
    
    L1x = 53.17;
    L1z = 8;
    L2  = 101.88;
    L3  = 149.16;

    theta1 = atan2(yL,xL);

    C1  = cos(theta1);
    S1  = sin(theta1);

    C3_temp = ( ( xL - L1x*C1 )^2 + ( yL - L1x*S1 )^2 + ( zL - L1z )^2 - L2^2 - L3^2 )/( 2*L2*L3 );
        
    if C3_temp>1
        C3 = 1;
    elseif C3_temp<-1
        C3 = -1;
    else
        C3 = C3_temp;
    end
    
    S3 = -sqrt((1 - C3^2));

    theta2 = atan2( zL-L1z, sqrt( (xL-L1x*C1)^2 + (yL - L1x*S1)^2 ) ) - atan2(L3*S3, L2 + L3*C3);

    theta3 = atan2(S3, C3);
    
end

== matlab function ForwardKinematicsSim2/leg 5/MATLAB Function1 ==
  data: theta1 input; Px2 output; theta2 input; Py2 output; Pz2 output
function [Px2,Py2,Pz2] = fcn(theta1,theta2)

    % Link lengths as defined in Figure 5.3
    L1x = 53.17;
    L1z = 8;
    L2  = 101.88;

    
    % Transformation from servo angles to end effector positions as given in
    % Equation 5.30
    C1  = cos(theta1);
    S1  = sin(theta1);
    C2  = cos(theta2);
    S2  = sin(theta2);
    
    H01 = [C1,  0,  S1, C1*L1x;...
           S1,  0, -C1, S1*L1x;...
            0,  1,   0,    L1z;...
            0,  0,   0,     1];
   
    H12 = [C2, -S2,  0, L2*C2;...
           S2,  C2,  0, L2*S2;...
            0,   0,  1,     0;...
            0,   0,  0,     1];  
    
    H02 = H01*H12;
 
Px2 = H02(1,4);Py2 = H02(2,4);Pz2 = H02(3,4);

== matlab function ForwardKinematicsSim2/leg 5/MATLAB Function2 ==
  data: theta1 input; Px1 output; Py1 output; Pz1 output
function [Px1,Py1,Pz1] = fcn(theta1)

    % Link lengths as defined in Figure 5.3
    L1x = 53.17;
    L1z = 8;

    % Transformation from servo angles to end effector positions as given in
    % Equation 5.30
    C1  = cos(theta1);
    S1  = sin(theta1);

    H01 = [C1,  0,  S1, C1*L1x;...
           S1,  0, -C1, S1*L1x;...
            0,  1,   0,    L1z;...
            0,  0,   0,     1];
 
Px1 = H01(1,4);Py1 = H01(2,4);Pz1 = H01(3,4);

== matlab function ForwardKinematicsSim2/leg 6/Forward Kinemat ==
  data: theta1 input; Px output; theta2 input; theta3 input; Py output; Pz output
function [Px,Py,Pz] = fcn(theta1,theta2,theta3)

    % degrees to radians
    d2r = pi/180;

    % Link lengths as defined in Figure 5.3
    L1x = 53.17;
    L1z = 8;
    L2  = 101.88;
    L3  = 149.16;

    % Transformation from servo angles to end effector positions as given in
    % Equation 5.30
    C1  = cos(theta1);
    S1  = sin(theta1);
    C2  = cos(theta2);
    S2  = sin(theta2);
    C23 = cos(theta2 + theta3);
    S23 = sin(theta2 + theta3);

    T03 = [C1*C23, -C1*S23,  S1, C1*(L1x + L3*C23 + L2*C2);...
            S1*C23, -S1*S23, -C1, S1*(L1x + L3*C23 + L2*C2);...
            S23,     C23,   0, L1z + L3*S23 + L2*S2;...
            0,       0,   0, 1];
 
Px = T03(1,4);Py = T03(2,4);Pz = T03(3,4);

== matlab function ForwardKinematicsSim2/leg 1/Forward Kinemat ==
  data: theta1 input; Px output; theta2 input; theta3 input; Py output; Pz output
function [Px,Py,Pz] = fcn(theta1,theta2,theta3)

    % degrees to radians
    d2r = pi/180;

    % Link lengths as defined in Figure 5.3
    L1x = 53.17;
    L1z = 8;
    L2  = 101.88;
    L3  = 149.16;

    % Transformation from servo angles to end effector positions as given in
    % Equation 5.30
    C1  = cos(theta1);
    S1  = sin(theta1);
    C2  = cos(theta2);
    S2  = sin(theta2);
    C23 = cos(theta2 + theta3);
    S23 = sin(theta2 + theta3);

    T03 = [C1*C23, -C1*S23,  S1, C1*(L1x + L3*C23 + L2*C2);...
            S1*C23, -S1*S23, -C1, S1*(L1x + L3*C23 + L2*C2);...
            S23,     C23,   0, L1z + L3*S23 + L2*S2;...
            0,       0,   0, 1];
 
Px = T03(1,4);Py = T03(2,4);Pz = T03(3,4);

== matlab function ForwardKinematicsSim2/leg 6/Inverse Kinematics ==
  data: xL input; theta1 output; yL input; zL input; theta2 output; theta3 output
function [theta1,theta2,theta3] = fcn(xL,yL,zL)
    
    L1x = 53.17;
    L1z = 8;
    L2  = 101.88;
    L3  = 149.16;

    theta1 = atan2(yL,xL);

    C1  = cos(theta1);
    S1  = sin(theta1);

    C3_temp = ( ( xL - L1x*C1 )^2 + ( yL - L1x*S1 )^2 + ( zL - L1z )^2 - L2^2 - L3^2 )/( 2*L2*L3 );

    if C3_temp>1
        C3 = 1;
    elseif C3_temp<-1
        C3 = -1;
    else
        C3 = C3_temp;
    end

    S3 = -sqrt((1 - C3^2));

    theta2 = atan2( zL-L1z, sqrt( (xL-L1x*C1)^2 + (yL - L1x*S1)^2 ) ) - atan2(L3*S3, L2 + L3*C3);

    theta3 = atan2(S3, C3);
    
end

== matlab function ForwardKinematicsSim2/leg 6/MATLAB Function1 ==
  data: theta1 input; Px2 output; theta2 input; Py2 output; Pz2 output
function [Px2,Py2,Pz2] = fcn(theta1,theta2)

    % Link lengths as defined in Figure 5.3
    L1x = 53.17;
    L1z = 8;
    L2  = 101.88;

    
    % Transformation from servo angles to end effector positions as given in
    % Equation 5.30
    C1  = cos(theta1);
    S1  = sin(theta1);
    C2  = cos(theta2);
    S2  = sin(theta2);
    
    H01 = [C1,  0,  S1, C1*L1x;...
           S1,  0, -C1, S1*L1x;...
            0,  1,   0,    L1z;...
            0,  0,   0,     1];
   
    H12 = [C2, -S2,  0, L2*C2;...
           S2,  C2,  0, L2*S2;...
            0,   0,  1,     0;...
            0,   0,  0,     1];  
    
    H02 = H01*H12;
 
Px2 = H02(1,4);Py2 = H02(2,4);Pz2 = H02(3,4);

== matlab function ForwardKinematicsSim2/leg 6/MATLAB Function2 ==
  data: theta1 input; Px1 output; Py1 output; Pz1 output
function [Px1,Py1,Pz1] = fcn(theta1)

    % Link lengths as defined in Figure 5.3
    L1x = 53.17;
    L1z = 8;

    % Transformation from servo angles to end effector positions as given in
    % Equation 5.30
    C1  = cos(theta1);
    S1  = sin(theta1);

    H01 = [C1,  0,  S1, C1*L1x;...
           S1,  0, -C1, S1*L1x;...
            0,  1,   0,    L1z;...
            0,  0,   0,     1];
 
Px1 = H01(1,4);Py1 = H01(2,4);Pz1 = H01(3,4);

== matlab function ForwardKinematicsSim2/leg 1/MATLAB Function2 ==
  data: theta1 input; Px1 output; Py1 output; Pz1 output
function [Px1,Py1,Pz1] = fcn(theta1)

    % Link lengths as defined in Figure 5.3
    L1x = 53.17;
    L1z = 8;

    % Transformation from servo angles to end effector positions as given in
    % Equation 5.30
    C1  = cos(theta1);
    S1  = sin(theta1);

    H01 = [C1,  0,  S1, C1*L1x;...
           S1,  0, -C1, S1*L1x;...
            0,  1,   0,    L1z;...
            0,  0,   0,     1];
 
Px1 = H01(1,4);Py1 = H01(2,4);Pz1 = H01(3,4);

== matlab function ForwardKinematicsSim2/leg 1/Inverse Kinematics ==
  data: xL input; theta1 output; yL input; zL input; theta2 output; theta3 output
function [theta1,theta2,theta3] = fcn(xL,yL,zL)
    
    L1x = 53.17;
    L1z = 8;
    L2  = 101.88;
    L3  = 149.16;

    theta1 = atan2(yL,xL);

    C1  = cos(theta1);
    S1  = sin(theta1);

    C3_temp = ( ( xL - L1x*C1 )^2 + ( yL - L1x*S1 )^2 + ( zL - L1z )^2 - L2^2 - L3^2 )/( 2*L2*L3 );
    
    if C3_temp>1
        C3 = 1;
    elseif C3_temp<-1
        C3 = -1;
    else
        C3 = C3_temp;
    end
    
    
    S3 = -sqrt((1 - C3^2));

    theta2 = atan2( zL-L1z, sqrt( (xL-L1x*C1)^2 + (yL - L1x*S1)^2 ) ) - atan2(L3*S3, L2 + L3*C3);

    theta3 = atan2(S3, C3);
    
end

== matlab function ForwardKinematicsSim2/leg 2/Forward Kinemat ==
  data: theta1 input; Px output; theta2 input; theta3 input; Py output; Pz output
function [Px,Py,Pz] = fcn(theta1,theta2,theta3)

    % degrees to radians
    d2r = pi/180;

    % Link lengths as defined in Figure 5.3
    L1x = 53.17;
    L1z = 8;
    L2  = 101.88;
    L3  = 149.16;

    % Transformation from servo angles to end effector positions as given in
    % Equation 5.30
    C1  = cos(theta1);
    S1  = sin(theta1);
    C2  = cos(theta2);
    S2  = sin(theta2);
    C23 = cos(theta2 + theta3);
    S23 = sin(theta2 + theta3);

    T03 = [C1*C23, -C1*S23,  S1, C1*(L1x + L3*C23 + L2*C2);...
            S1*C23, -S1*S23, -C1, S1*(L1x + L3*C23 + L2*C2);...
            S23,     C23,   0, L1z + L3*S23 + L2*S2;...
            0,       0,   0, 1];
 
Px = T03(1,4);Py = T03(2,4);Pz = T03(3,4);

== matlab function ForwardKinematicsSim2/leg 2/Inverse Kinematics ==
  data: xL input; theta1 output; yL input; zL input; theta2 output; theta3 output
function [theta1,theta2,theta3] = fcn(xL,yL,zL)
    
    L1x = 53.17;
    L1z = 8;
    L2  = 101.88;
    L3  = 149.16;

    theta1 = atan2(yL,xL);

    C1  = cos(theta1);
    S1  = sin(theta1);

    C3_temp = ( ( xL - L1x*C1 )^2 + ( yL - L1x*S1 )^2 + ( zL - L1z )^2 - L2^2 - L3^2 )/( 2*L2*L3 );
    
    if C3_temp>1
        C3 = 1;
    elseif C3_temp<-1
        C3 = -1;
    else
        C3 = C3_temp;
    end
    
    S3 = -sqrt((1 - C3^2));

    theta2 = atan2( zL-L1z, sqrt( (xL-L1x*C1)^2 + (yL - L1x*S1)^2 ) ) - atan2(L3*S3, L2 + L3*C3);

    theta3 = atan2(S3, C3);
    
end

== matlab function ForwardKinematicsSim2/leg 2/MATLAB Function1 ==
  data: theta1 input; Px2 output; theta2 input; Py2 output; Pz2 output
function [Px2,Py2,Pz2] = fcn(theta1,theta2)

    % Link lengths as defined in Figure 5.3
    L1x = 53.17;
    L1z = 8;
    L2  = 101.88;

    
    % Transformation from servo angles to end effector positions as given in
    % Equation 5.30
    C1  = cos(theta1);
    S1  = sin(theta1);
    C2  = cos(theta2);
    S2  = sin(theta2);
    
    H01 = [C1,  0,  S1, C1*L1x;...
           S1,  0, -C1, S1*L1x;...
            0,  1,   0,    L1z;...
            0,  0,   0,     1];
   
    H12 = [C2, -S2,  0, L2*C2;...
           S2,  C2,  0, L2*S2;...
            0,   0,  1,     0;...
            0,   0,  0,     1];  
    
    H02 = H01*H12;
 
Px2 = H02(1,4);Py2 = H02(2,4);Pz2 = H02(3,4);

== matlab function ForwardKinematicsSim2/leg 2/MATLAB Function2 ==
  data: theta1 input; Px1 output; Py1 output; Pz1 output
function [Px1,Py1,Pz1] = fcn(theta1)

    % Link lengths as defined in Figure 5.3
    L1x = 53.17;
    L1z = 8;

    % Transformation from servo angles to end effector positions as given in
    % Equation 5.30
    C1  = cos(theta1);
    S1  = sin(theta1);

    H01 = [C1,  0,  S1, C1*L1x;...
           S1,  0, -C1, S1*L1x;...
            0,  1,   0,    L1z;...
            0,  0,   0,     1];
 
Px1 = H01(1,4);Py1 = H01(2,4);Pz1 = H01(3,4);

== matlab function ForwardKinematicsSim2/leg 3/Forward Kinemat ==
  data: theta1 input; Px output; theta2 input; theta3 input; Py output; Pz output
function [Px,Py,Pz] = fcn(theta1,theta2,theta3)

    % degrees to radians
    d2r = pi/180;

    % Link lengths as defined in Figure 5.3
    L1x = 53.17;
    L1z = 8;
    L2  = 101.88;
    L3  = 149.16;

    % Transformation from servo angles to end effector positions as given in
    % Equation 5.30
    C1  = cos(theta1);
    S1  = sin(theta1);
    C2  = cos(theta2);
    S2  = sin(theta2);
    C23 = cos(theta2 + theta3);
    S23 = sin(theta2 + theta3);

    T03 = [C1*C23, -C1*S23,  S1, C1*(L1x + L3*C23 + L2*C2);...
            S1*C23, -S1*S23, -C1, S1*(L1x + L3*C23 + L2*C2);...
            S23,     C23,   0, L1z + L3*S23 + L2*S2;...
            0,       0,   0, 1];
 
Px = T03(1,4);Py = T03(2,4);Pz = T03(3,4);
